simulink subsystem "Transfer_fcn_plant"  (R2022b)
settings: Solver=VariableStepAuto  StartTime=0.0  StopTime=10.0  RelTol=1e-3
values from neighbouring files (symbols this model uses):
  plant_den : value not decoded    [control_system_data.sldd]
  plant_num : value not decoded    [control_system_data.sldd]
settings Model: DefaultTestHarness=Transfer_fcn_plant_test_1  Creator=tshintai  LastModifiedBy=tshintai
settings DebuggingCC: UnconnectedInputMsg=warning  UnconnectedOutputMsg=warning  UnconnectedLineMsg=warning
settings ModelReferenceCC: EnableRefExpFcnMdlSchedulingChecks=on
settings RTWCC: DLArmComputeVersion=19.05

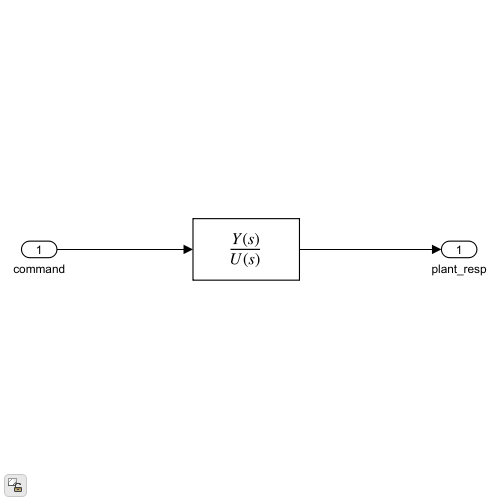
[thumbnail: Simulink's stored preview of the top-level diagram]
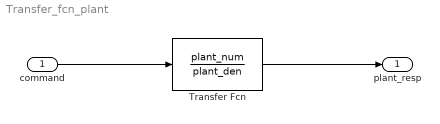
== system Transfer_fcn_plant ==
  command : Inport
  Transfer Fcn : TransferFcn  Numerator=plant_num  Denominator=plant_den
  plant_resp : Outport
  wires:
  command/1 -> Transfer Fcn/1
  Transfer Fcn/1 -> plant_resp/1
